simulink model "c221007_FCEV_CDCS"  (R2022b)
settings: Solver=ode4  StartTime=1  StopTime=size(Driving_cycle_v_kmph,1)  FixedStep=Auto  RelTol=1e-3  EnableMultiTasking=on
values from neighbouring files (symbols this model uses):
  Bat_eff_chg_average = 0.969    [FCEV_original_data.mat]
  Bat_eff_dis_average = 0.9632    [FCEV_original_data.mat]
  Bat_end_of_life_percent = 20    [FCEV_original_data.mat]
  Bat_I_chg_max = -120    [FCEV_original_data.mat]
  Bat_I_dis_max = 200    [FCEV_original_data.mat]
  Bat_nom_Ic = 2.5    [FCEV_original_data.mat]
  Bat_nom_SOC = 0.35    [FCEV_original_data.mat]
  Bat_nom_temp_oC = 25    [FCEV_original_data.mat]
  Bat_num_pa = 9    [FCEV_original_data.mat]
  Bat_num_se = 97    [FCEV_original_data.mat]
  Bat_ori_C1_chg_F = [397.526659684 455.660832136 435.08783522 460.845064365 457.605812374 417.289828504 416.373906992 359.741413056 321.561704819 1109.14132554 1165.67733205 1135.97600211 ... (72 elements, 9x8)]    [FCEV_original_data.mat]
  Bat_ori_C1_dis_F = [187.121968588 287.083505726 346.448009002 395.529439835 387.517274826 389.973134196 432.856765051 486.92921923 512.158935268 425.990733989 614.68708868 771.472592368 ... (72 elements, 9x8)]    [FCEV_original_data.mat]
  Bat_ori_C2_chg_F = [8748.48589695 7773.35875681 9404.86567646 8934.73981058 8290.58671366 7592.78422269 7759.44623103 7396.59043829 6151.35152293 16187.7227039 11721.8480541 13157.8579836 ... (72 elements, 9x8)]    [FCEV_original_data.mat]
  Bat_ori_C2_dis_F = [2939.81325553 4590.73311898 5504.93546413 5887.5077374 6534.37836712 7765.46899768 10584.7751706 10372.0508438 9238.72693885 5207.86390693 7911.43744944 8879.62137571 ... (72 elements, 9x8)]    [FCEV_original_data.mat]
  Bat_ori_cap_max_Ah = 20.7    [Config_c221218.m]    (also in Config_c230117.m; Config_c230321.m; FCEV_original_data.mat)
  Bat_ori_dUdt4 = [-0.303773584906 -0.249056603774 -0.115094339623 -0.0396226415094 0.0396226415094 0.0641509433962 0.107547169811 0.111320754717 0.0415094339623 0.0547169811321 0.130188679245]    [FCEV_original_data.mat]
  Bat_ori_R0_chg_O = [0.0771669453735 0.0731809311402 0.0726556782939 0.0729965156794 0.0731758310684 0.0742031005051 0.0721266921026 0.0714211058078 0.0714186176143 0.0374124505155 0.0354566732504 0.0345430657188 ... (72 elements, 9x8)]    [FCEV_original_data.mat]
  Bat_ori_R0_dis_O = [0.0819458671157 0.0812429476608 0.0803749674507 0.0805513601722 0.0838629023857 0.0850797840015 0.0829875518672 0.0826388888889 0.0812514106148 0.0428124986417 0.0424658903711 0.0428572670451 ... (72 elements, 9x8)]    [FCEV_original_data.mat]
  Bat_ori_R1_chg_O = [0.114339870884 0.105392753268 0.104421193553 0.109821896183 0.114868279838 0.123333154908 0.129174812826 0.149917249373 0.174896487845 0.0420560161846 0.0390948352938 0.0370122837364 ... (72 elements, 9x8)]    [FCEV_original_data.mat]
  Bat_ori_R1_dis_O = [0.304806399643 0.213604089624 0.171463520004 0.151183840498 0.140630862434 0.128795299077 0.116857791733 0.112567113582 0.106368362501 0.0943235089866 0.0730697254134 0.0611414736086 ... (72 elements, 9x8)]    [FCEV_original_data.mat]
  Bat_ori_R2_chg_O = [0.134518959939 0.17565045702 0.161100627268 0.189032232545 0.205639040497 0.226170473035 0.223651875822 0.181765694192 0.212966950836 0.073628872144 0.0788540822416 0.0792414571734 ... (72 elements, 9x8)]    [FCEV_original_data.mat]
  Bat_ori_R2_dis_O = [0.354968099904 0.285293035102 0.286338708953 0.298763853987 0.248762838155 0.178586175471 0.129047399775 0.188406991173 0.174494800676 0.131839238891 0.123225430215 0.132069033134 ... (72 elements, 9x8)]    [FCEV_original_data.mat]
  Bat_ori_SOC2 = [0 0.001 0.002 0.003 0.004 0.005 0.006 0.007 0.008 0.009 0.01 0.011 ... (1001 elements, 1x1001)]    [FCEV_original_data.mat]
  Bat_ori_SOC4 = [-0.00598301069999 0.0920117618231 0.190864167279 0.289083557951 0.387343788287 0.485011843502 0.5850485992 0.678163031937 0.774810095565 0.876684636119 0.972739524626]    [FCEV_original_data.mat]
  Bat_ori_Uoc_chg_V = [2.4478 2.54923264342 2.6007 2.6383 2.66953057366 2.69636321708 2.7197 2.74042850391 2.75906114733 2.77619379074 2.792 2.80675907757 ... (1001 elements, 1x1001)]    [FCEV_original_data.mat]
  Bat_ori_Uoc_dis_V = [1.9998 2.03916768329 2.24724374236 2.39700902919 2.48767431602 2.5476 2.5882 2.6202 2.64771773167 2.6719 2.6933 2.71251566192 ... (1001 elements, 1x1001)]    [FCEV_original_data.mat]
  Bat_ori_Uoc_V = [2.2238 2.29420016335 2.42397187118 2.5176545146 2.57860244484 2.62198160854 2.65395 2.68031425195 2.7033894395 2.72404689537 2.74265 2.75963736975 ... (1001 elements, 1x1001)]    [FCEV_original_data.mat]
  Bat_single_capacity_nom_Ah = 2.3    [FCEV_original_data.mat]
  Bat_SOC_cs_max = 0.4    [FCEV_original_data.mat]
  Bat_SOC_cs_min = 0.2    [FCEV_original_data.mat]
  Bat_SOC_ini = 0.3    [Config_c22100601.m]    (also in Config_c22100701.m; FCEV_original_data.mat = 0.45)
  Bat_SOC_max = 0.9    [FCEV_original_data.mat]
  Bat_SOC_min = 0.3    [FCEV_original_data.mat]
  Bat_temp_amb_oC = 25    [FCEV_original_data.mat]
  Bat_temp_cool_oC = 25    [FCEV_original_data.mat]
  Bat_U_avg_V = Bat_num_se*mean(Bat_ori_Uoc_V)    [Config_c22100601.m]    (also in Config_c22100701.m)
  DCAC_eff = 0.95    [FCEV_original_data.mat]
  DCDC_ori_eff = [0.95 0.96 0.97 0.976 0.98 0.978 0.973 0.962]    [FCEV_original_data.mat]
  DCDC_ori_power_kW = [0 10 20 30 40 50 60 70]    [FCEV_original_data.mat]
  FC_fuel_mass_ini_kg = 10    [FCEV_original_data.mat]
  FC_ori_eff = [0.1 0.33 0.492 0.533 0.559 0.596 0.591 0.562 0.508]    [FCEV_original_data.mat]
  FC_ori_fuel_rate_gps = [0 0.0505050505051 0.0846883468835 0.117260787992 0.149075730471 0.279642058166 0.423011844332 0.593119810202 0.820209973753]    [FCEV_original_data.mat]
  FC_ori_power_kW = [0 2 5 7.5 10 20 30 40 50]    [FCEV_original_data.mat]
  FC_power_max_kW = 50    [FCEV_original_data.mat]
  FC_power_min_kW = 0    [FCEV_original_data.mat]
  MC_eff_brk_average = 0.810578512397    [FCEV_original_data.mat]
  MC_eff_dri_average = 0.810578512397    [FCEV_original_data.mat]
  MC_inertia = 0.06    [FCEV_original_data.mat]
  MC_ori_eff = [0.7 0.78 0.85 0.86 0.81 0.82 0.79 0.78 0.78 0.78 0.78 0.7 ... (231 elements, 11x21)]    [FCEV_original_data.mat]
  MC_ori_power_brk_req_kW = [0 -28.3912930389 -56.7825860779 -85.1738791168 -113.565172156 -141.956465195 -170.347758234 -198.739051273 -227.130344311 -255.52163735 -283.912930389 0 ... (121 elements, 11x11)]    [FCEV_original_data.mat]
  MC_ori_power_dri_req_kW = [0 0 0 0 0 0 0 0 0 0 0 0 ... (121 elements, 11x11)]    [FCEV_original_data.mat]
  MC_ori_spd_rpm = [0 1000 2000 3000 4000 5000 6000 7000 8000 9000 10000]    [FCEV_original_data.mat]
  MC_ori_trq_brk_max_Nm = [-271.1368 -271.1368 -271.1368 -237.5159 -178.1369 -142.4824 -118.7579 -101.8119 -89.0685 -79.172 -71.1734]    [FCEV_original_data.mat]
  MC_ori_trq_brk_Nm = [-271.136848522 -244.02316367 -216.909478817 -189.795793965 -162.682109113 -135.568424261 -108.454739409 -81.3410545565 -54.2273697044 -27.1136848522 0]    [FCEV_original_data.mat]
  MC_ori_trq_dri_max_Nm = [271.1368 271.1368 271.1368 237.5159 178.1369 142.4824 118.7579 101.8119 89.0685 79.172 71.1734]    [FCEV_original_data.mat]
  MC_ori_trq_dri_Nm = [0 27.1136848522 54.2273697044 81.3410545565 108.454739409 135.568424261 162.682109113 189.795793965 216.909478817 244.02316367 271.136848522]    [FCEV_original_data.mat]
  MC_ori_trq_Nm = [-271.136848522 -244.02316367 -216.909478817 -189.795793965 -162.682109113 -135.568424261 -108.454739409 -81.3410545565 -54.2273697044 -27.1136848522 0 27.1136848522 ... (21 elements, 1x21)]    [FCEV_original_data.mat]
  MC_power_max_kW = 75    [FCEV_original_data.mat]
  MC_spd_max_rpm = 10000    [FCEV_original_data.mat]
  MC_spd_min_rpm = 0    [FCEV_original_data.mat]
  MC_spd_scale = 1    [FCEV_original_data.mat]
  MC_trq_scale = 1    [FCEV_original_data.mat]
  MC_U_min_V = 120    [FCEV_original_data.mat]
  Road_u = 0.75    [FCEV_original_data.mat]
  S_r = floor(max(Sr_SOC_process(:,1))):-1:0    [Config_c22100601.m]    (also in Config_c22100701.m)
  Time_sample = 60    [Driving_cycle_recognition_data.mat]
  Trip_distance_total_km = sum(Driving_cycle_v_kmph(:,2)/3.6)/1000    [Config_c22100601.m]    (also in Config_c22100701.m)
  usd2rmb = 7.116    [Config_c22100601.m]    (also in Config_c22100701.m; Config_c221106.m = 6; Config_c221112.m = 6; Config_c221127.m = 6)
  Veh_air_density_kgpm2 = 1.2    [FCEV_original_data.mat]
  Veh_brk_front = [1 0.6 0.608 0.61 0.618 0.624 0.636 0.645 0.655]    [FCEV_original_data.mat]
  Veh_brk_z = [0.1 0.2 0.3 0.4 0.5 0.6 0.7 0.8 0.9]    [FCEV_original_data.mat]
  Veh_brk_z_max = 0.7    [FCEV_original_data.mat]
  Veh_brk_z_min = 0.1    [FCEV_original_data.mat]
  Veh_coeff_drag = 0.312    [FCEV_original_data.mat]
  Veh_coeff_roll = 0.00863    [FCEV_original_data.mat]
  Veh_final_drive_inertia = 0.1105    [FCEV_original_data.mat]
  Veh_final_drive_ratio = 3.47    [FCEV_original_data.mat]
  Veh_frontal_area_m2 = 2.06    [FCEV_original_data.mat]
  Veh_gravity_acc_ms2 = 9.81    [FCEV_original_data.mat]
  Veh_mass_cargo_kg = 113    [FCEV_original_data.mat]
  Veh_mass_curb_kg = 1157    [FCEV_original_data.mat]
  Veh_mech_eff = 0.9    [FCEV_original_data.mat]
  Veh_rotary_mass_conversion_factor = 1.05    [FCEV_original_data.mat]
  Veh_size_cg_height_m = 0.53    [FCEV_original_data.mat]
  Veh_wheel_inertia = 3.1039    [FCEV_original_data.mat]
  Veh_wheel_radius_m = 0.313    [FCEV_original_data.mat]
  Veh_wt_frac_front = 0.5    [FCEV_original_data.mat]
undefined symbols (not defined in the file or in its folder): alpha, Bat_ori_temp, Sr_e
libraries: neural x10
(part 2 of 5)

== system c221007_FCEV_CDCS/整车动力学模型/加速阻力 ==
  车速 km/h : Inport
  Add : Sum  Inputs=+-
  Add1 : Sum  Inputs=+-
  Add2 : Sum
  Clock : Clock
  Constant : Constant  Value=0
  Constant1 : Constant  Value=Veh_rotary_mass_conversion_factor
  Constant2 : Constant  Value=Veh_mass_curb_kg
  Constant3 : Constant  Value=Veh_mass_cargo_kg
  Divide : Product  Inputs=***/
  Fj : Scope
  Gain : Gain
  Memory : Memory  InheritSampleTime=on
  Memory1 : Memory
  Saturation : Saturate  UpperLimit=1.1  LowerLimit=0.9
  Switch : Switch  Criteria=u2 > Threshold  SaturateOnIntegerOverflow=off  InputSameDT=off
  km/h->m/s : Gain  Gain=1/3.6
  加速阻力 N : Outport
  wires:
  车速 km/h/1 -> Memory/1, Add/1
  Add/1 -> km/h->m/s/1
  km/h->m/s/1 -> Switch/2, Divide/2
  Gain/1 -> 加速阻力 N/1, Fj/1
  Memory/1 -> Add/2
  Memory1/1 -> Add1/2
  Add2/1 -> Divide/1
  Constant2/1 -> Add2/1
  Constant3/1 -> Add2/2
  Constant1/1 -> Divide/3
  Clock/1 -> Memory1/1, Add1/1
  Divide/1 -> Switch/1
  Constant/1 -> Switch/3
  Switch/1 -> Gain/1
  Add1/1 -> Saturation/1
  Saturation/1 -> Divide/4

== system c221007_FCEV_CDCS/整车动力学模型/坡道阻力 ==
  车辆平均车速1 : Inport
  预测坡度 : Inport  Port=2
  Add : Sum  Inputs=+-
  Add1 : Sum
  Constant : Constant  Value=0
  Constant1 : Constant  Value=Veh_mass_cargo_kg
  Constant2 : Constant  Value=Veh_mass_curb_kg
  Constant3 : Constant  Value=Veh_gravity_acc_ms2
  Fi : Scope
  Memory : Memory  InheritSampleTime=on
  Product : Product  Inputs=3  RndMeth=Zero
  Switch : Switch  SaturateOnIntegerOverflow=off  InputSameDT=off
  Switch1 : Switch  Criteria=u2 > Threshold  SaturateOnIntegerOverflow=off  InputSameDT=off
  Trigonometric Function : Trigonometry  Operator=atan
  Trigonometric Function1 : Trigonometry
  坡道阻力 N : Outport
  wires:
  Trigonometric Function/1 -> Trigonometric Function1/1
  Trigonometric Function1/1 -> Product/1
  Constant3/1 -> Product/3
  Constant/1 -> Switch/3, Switch1/3
  预测坡度/1 -> Trigonometric Function/1
  Switch1/1 -> 坡道阻力 N/1, Fi/1
  Add1/1 -> Product/2
  Constant2/1 -> Add1/1
  Constant1/1 -> Add1/2
  车辆平均车速1/1 -> Add/1, Memory/1, Switch1/2
  Memory/1 -> Add/2
  Product/1 -> Switch/1
  Add/1 -> Switch/2
  Switch/1 -> Switch1/1

== system c221007_FCEV_CDCS/整车动力学模型/滚动阻力 ==
  车辆平均车速 km/h : Inport
  预测坡度 : Inport  Port=2
  "  1" : Constant  Value=Veh_coeff_roll
  Add : Sum  Inputs=+-
  Add1 : Sum
  Constant : Constant  Value=0
  Constant1 : Constant  Value=Veh_gravity_acc_ms2
  Constant2 : Constant  Value=Veh_mass_curb_kg
  Constant3 : Constant  Value=Veh_mass_cargo_kg
  Fcn1 : Fcn  Expr=atan(u)
  Fcn2 : Fcn  Expr=cos(u)
  Ff : Scope
  Memory : Memory  InheritSampleTime=on
  Product : Product  Inputs=4  RndMeth=Zero
  Switch : Switch  Criteria=u2 > Threshold  SaturateOnIntegerOverflow=off  InputSameDT=off
  Switch1 : Switch  SaturateOnIntegerOverflow=off  InputSameDT=off
  滚动阻力 N : Outport
  wires:
  Fcn2/1 -> Product/3
  Constant/1 -> Switch1/3, Switch/3
  Add1/1 -> Product/1
  Fcn1/1 -> Fcn2/1
  预测坡度/1 -> Fcn1/1
  Constant2/1 -> Add1/1
  Constant3/1 -> Add1/2
  车辆平均车速 km/h/1 -> Switch/2, Memory/1, Add/1
  Switch/1 -> Ff/1, 滚动阻力 N/1
  Constant1/1 -> Product/2
  "  1"/1 -> Product/4
  Product/1 -> Switch1/1
  Memory/1 -> Add/2
  Add/1 -> Switch1/2
  Switch1/1 -> Switch/1

== system c221007_FCEV_CDCS/整车动力学模型/空气阻力 ==
  veh_spd km/h : Inport
  Add : Sum  Inputs=-+
  Constant : Constant  Value=0
  Constant1 : Constant  Value=Veh_frontal_area_m2
  Constant2 : Constant  Value=Veh_coeff_drag
  Fw : Scope
  Gain : Gain  Gain=1/21.15
  Memory : Memory  InheritSampleTime=on
  Product : Product  Inputs=4  RndMeth=Zero
  Switch : Switch  SaturateOnIntegerOverflow=off  InputSameDT=off
  空气阻力 N : Outport
  wires:
  Constant1/1 -> Product/1
  Constant2/1 -> Product/2
  veh_spd km/h/1 -> Product/3, Memory/1, Add/2, Product/4
  Product/1 -> Gain/1
  Constant/1 -> Switch/3
  Gain/1 -> Switch/1
  Add/1 -> Switch/2
  Memory/1 -> Add/1
  Switch/1 -> Fw/1, 空气阻力 N/1

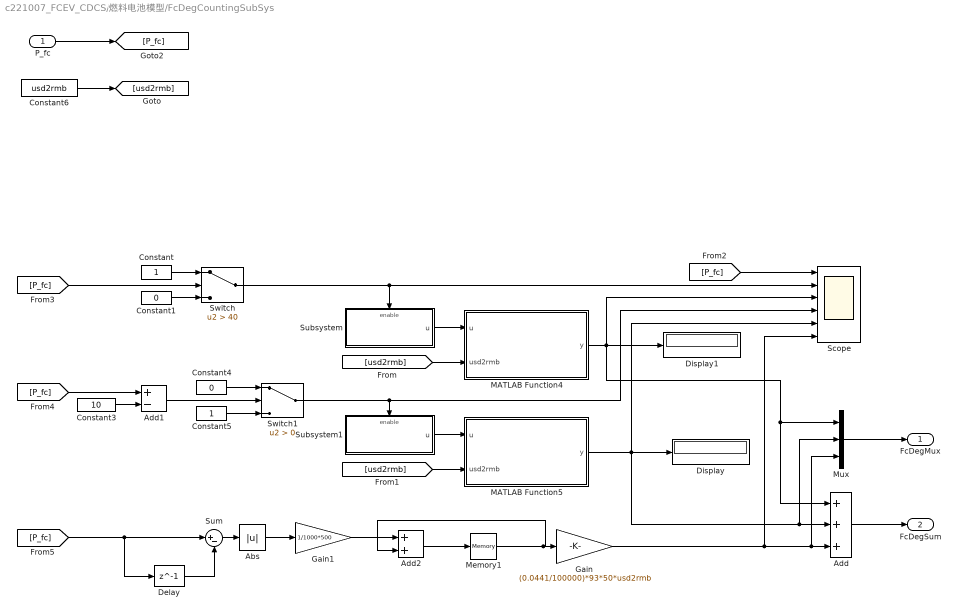
== system c221007_FCEV_CDCS/燃料电池模型/FcDegCountingSubSys ==
  P_fc : Inport
  Abs : Abs  SaturateOnIntegerOverflow=off
  Add : Sum  Inputs=+++
  Add1 : Sum  Inputs=+-
  Add2 : Sum
  Constant : Constant
  Constant1 : Constant  Value=0
  Constant3 : Constant  Value=10
  Constant4 : Constant  Value=0
  Constant5 : Constant
  Constant6 : Constant  Value=usd2rmb
  Delay : Delay  DelayLength=1
  Display : Display
  Display1 : Display
  Gain : Gain  Gain=(0.0441/100000)*93*50*usd2rmb
  Gain1 : Gain  Gain=1/1000*500
  MATLAB Function4 : MATLAB Function  TreatAsAtomicUnit=on
  MATLAB Function5 : MATLAB Function  TreatAsAtomicUnit=on
  Memory1 : Memory
  Mux : Mux  Inputs=3
  Scope : Scope  NumInputPorts=6
  Subsystem : Subsystem
  Subsystem1 : Subsystem
  Sum : Sum  Inputs=|+-
  Switch : Switch  Criteria=u2 > Threshold  Threshold=40  SaturateOnIntegerOverflow=off  InputSameDT=off
  Switch1 : Switch  Criteria=u2 > Threshold  SaturateOnIntegerOverflow=off  InputSameDT=off
  FcDegMux : Outport
  FcDegSum : Outport  Port=2
  wires:
  MATLAB Function5/1(y) -> Scope/5, Display/1, Mux/2, Add/2
  Constant3/1 -> Add1/2
  Constant5/1 -> Switch1/3
  Switch1/1 -> Scope/4, Subsystem1/Enable
  Add1/1 -> Switch1/2
  Subsystem/1(u) -> MATLAB Function4/1(u)
  Constant/1 -> Switch/1
  [usd2rmb] -> MATLAB Function4/2(usd2rmb)
  Constant1/1 -> Switch/3
  Constant4/1 -> Switch1/1
  [usd2rmb] -> MATLAB Function5/2(usd2rmb)
  Switch/1 -> Scope/2, Subsystem/Enable
  P_fc/1 -> [P_fc]
  Subsystem1/1(u) -> MATLAB Function5/1(u)
  MATLAB Function4/1(y) -> Scope/3, Mux/1, Add/1, Display1/1
  Constant6/1 -> [usd2rmb]
  [P_fc] -> Scope/1
  Gain/1 -> Scope/6, Mux/3, Add/3
  Gain1/1 -> Add2/1
  Add2/1 -> Memory1/1
  Sum/1 -> Abs/1
  Abs/1 -> Gain1/1
  Delay/1 -> Sum/2
  Memory1/1 -> Gain/1, Add2/2
  [P_fc] -> Delay/1, Sum/1
  [P_fc] -> Switch/2
  [P_fc] -> Add1/1
  Add/1 -> FcDegSum/1
  Mux/1 -> FcDegMux/1

== system c221007_FCEV_CDCS/燃料电池模型/Fuel Rate Calculation1 ==
  note: Transient load response
  fc pwr : Inport
  "FC hydrogen consumption rate " : Lookup_n-D  NumberOfTableDimensions=1  BreakpointsForDimension1=FC_ori_power_kW  Table=FC_ori_fuel_rate_gps  RndMeth=Simplest
  fcv_H2_rate (g/s)1 : Outport
  wires:
  fc pwr/1 -> "FC hydrogen consumption rate "/1
  "FC hydrogen consumption rate "/1 -> fcv_H2_rate (g/s)1/1  "fcv_hot_H2_hist"

== system c221007_FCEV_CDCS/燃料电池模型/Fuel cell efficiency calculation ==
  note: Transient load response
  fc power : Inport
  "FC efficiency " : Lookup_n-D  NumberOfTableDimensions=1  BreakpointsForDimension1=FC_ori_power_kW  Table=FC_ori_eff  RndMeth=Simplest
  "fc_eff " : Outport
  wires:
  "FC efficiency "/1 -> "fc_eff "/1
  fc power/1 -> "FC efficiency "/1

== system c221007_FCEV_CDCS/燃料电池模型/Power Calculation ==
  note: Transient load response
  fc on : Inport
  Power command (kW) : Inport  Port=2
  "   " : Constant  Value=0
  Switch2 : Switch  Threshold=0.5
  Power output (kW) : Outport
  wires:
  "   "/1 -> Switch2/3
  Power command (kW)/1 -> Switch2/1
  fc on/1 -> Switch2/2
  Switch2/1 -> Power output (kW)/1

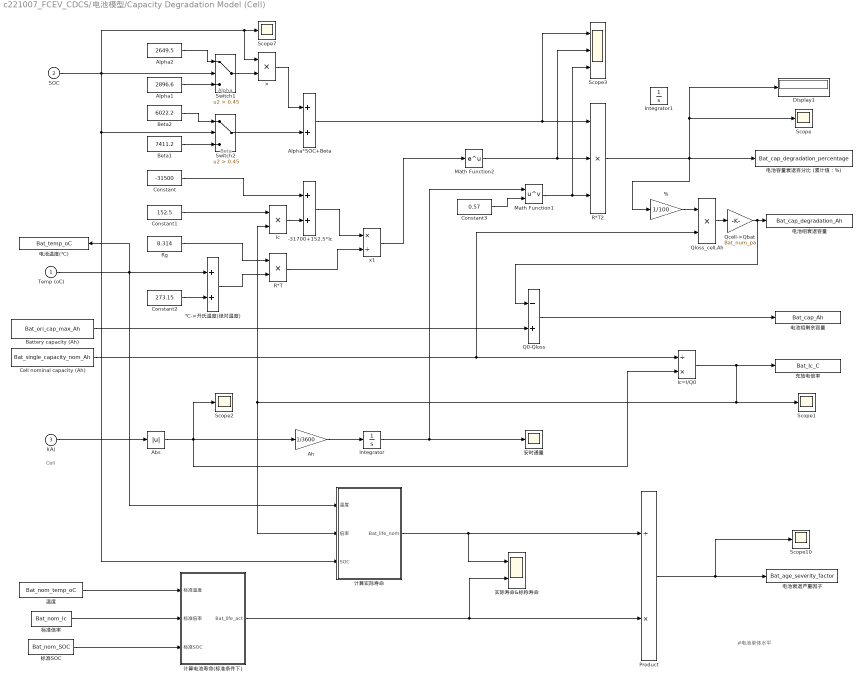
== system c221007_FCEV_CDCS/电池模型/Capacity Degradation Model (Cell) ==
  note: Cell
  note: #电池单体水平
  note: Beta
  note: Alpha
  Temp (oC) : Inport
  SOC : Inport  Port=2
  I(A) : Inport  Port=3
  % : Gain  Gain=1/100
  -31700+152.5*Ic : Sum  InputSameDT=on  SaturateOnIntegerOverflow=on  OutDataTypeStr=Inherit: Same as first input
  Abs : Abs  SaturateOnIntegerOverflow=off
  Ah : Gain  Gain=1/3600
  Alpha*SOC+Beta : Sum  InputSameDT=on  SaturateOnIntegerOverflow=on  OutDataTypeStr=Inherit: Same as first input
  Alpha1 : Constant  Value=2896.6
  Alpha2 : Constant  Value=2649.5
  Battery capacity (Ah) : Constant  Value=Bat_ori_cap_max_Ah
  Beta1 : Constant  Value=7411.2
  Beta2 : Constant  Value=6022.2
  Cell nominal capacity (Ah) : Constant  Value=Bat_single_capacity_nom_Ah
  Constant : Constant  Value=-31500
  Constant1 : Constant  Value=152.5
  Constant2 : Constant  Value=273.15
  Constant3 : Constant  Value=0.57
  Display1 : Display
  Ic : Product  InputSameDT=on  RndMeth=Zero  SaturateOnIntegerOverflow=on  OutDataTypeStr=Inherit: Same as first input
  Ic=I/Q0 : Product  Inputs=/*  InputSameDT=on  RndMeth=Zero  SaturateOnIntegerOverflow=on  OutDataTypeStr=Inherit: Same as first input
  Integrator : Integrator  InitialCondition=eps
  Integrator1 : Integrator
  Math Function1 : Math  Operator=pow  SignedPower=on
  Math Function2 : Math  SignedPower=on
  Product : Product  Inputs=/*
  Q0-Qloss : Sum  Inputs=-+  InputSameDT=on  SaturateOnIntegerOverflow=on  OutDataTypeStr=Inherit: Same as first input
  Qcell->Qbat : Gain  Gain=Bat_num_pa  SaturateOnIntegerOverflow=on  OutDataTypeStr=Inherit: Same as input  ParamDataTypeStr=Inherit: Same as input
  Qloss_cell,Ah : Product  InputSameDT=on  RndMeth=Zero  SaturateOnIntegerOverflow=on  OutDataTypeStr=Inherit: Same as first input
  R*T : Product  InputSameDT=on  RndMeth=Zero  SaturateOnIntegerOverflow=on  OutDataTypeStr=Inherit: Same as first input
  R*T2 : Product  Inputs=3  InputSameDT=on  RndMeth=Zero  SaturateOnIntegerOverflow=on  OutDataTypeStr=Inherit: Same as first input
  Rg : Constant  Value=8.314
  Scope{,1..2,7,10} (5 alike) : Scope
  Scope3 : Scope  NumInputPorts=3
  Switch1 : Switch  Criteria=u2 > Threshold  Threshold=0.45
  Switch2 : Switch  Criteria=u2 > Threshold  Threshold=0.45
  x1 : Product  Inputs=*/  InputSameDT=on  RndMeth=Zero  SaturateOnIntegerOverflow=on  OutDataTypeStr=Inherit: Same as first input
  × : Product  InputSameDT=on  RndMeth=Zero  SaturateOnIntegerOverflow=on  OutDataTypeStr=Inherit: Same as first input
  ℃->开氏温度(绝对温度) : Sum  InputSameDT=on  SaturateOnIntegerOverflow=on  OutDataTypeStr=Inherit: Same as first input
  充放电倍率 : ToWorkspace  VariableName=Bat_Ic_C  SampleTime=-1
  安时通量 : Scope
  实际寿命&标称寿命 : Scope  NumInputPorts=2
  标准SOC : Constant  Value=Bat_nom_SOC
  标准倍率 : Constant  Value=Bat_nom_Ic
  温度 : Constant  Value=Bat_nom_temp_oC  VectorParams1D=off
  电池容量衰退百分比 (累计值：%) : ToWorkspace  VariableName=Bat_cap_degradation_percentage  SampleTime=-1
  电池温度(℃) : ToWorkspace  VariableName=Bat_temp_oC  SampleTime=-1
  电池组剩余容量 : ToWorkspace  VariableName=Bat_cap_Ah  SampleTime=-1
  电池组衰退容量 : ToWorkspace  VariableName=Bat_cap_degradation_Ah  SampleTime=-1
  电池衰退严重因子 : ToWorkspace  VariableName=Bat_age_severity_factor  SampleTime=-1
  计算实际寿命 : Subsystem
  计算电池寿命(标准条件下) : Subsystem
  wires:
  SOC/1 -> Switch1/2, Scope7/1, ×/1, Switch2/2, 计算实际寿命/3(SOC)
  Alpha2/1 -> Switch1/1
  Alpha1/1 -> Switch1/3
  Beta2/1 -> Switch2/1
  Beta1/1 -> Switch2/3
  Switch1/1 -> ×/2
  Switch2/1 -> Alpha*SOC+Beta/2
  ×/1 -> Alpha*SOC+Beta/1
  Rg/1 -> R*T/1
  ℃->开氏温度(绝对温度)/1 -> R*T/2
  Ic=I/Q0/1 -> Scope1/1, Ic/2, 计算实际寿命/2(倍率), 充放电倍率/1
  Alpha*SOC+Beta/1 -> R*T2/1, Scope3/1
  Constant/1 -> -31700+152.5*Ic/1
  Ic/1 -> -31700+152.5*Ic/2
  Constant1/1 -> Ic/1
  -31700+152.5*Ic/1 -> x1/1
  R*T/1 -> x1/2
  Math Function2/1 -> R*T2/2, Scope3/2
  x1/1 -> Math Function2/1
  Math Function1/1 -> R*T2/3, Scope3/3
  R*T2/1 -> Scope/1, Display1/1, 电池容量衰退百分比 (累计值：%)/1, %/1
  Abs/1 -> Ic=I/Q0/2, Ah/1, Scope2/1
  Integrator/1 -> Math Function1/1, 安时通量/1
  Temp (oC)/1 -> 计算实际寿命/1(温度), 电池温度(℃)/1, ℃->开氏温度(绝对温度)/1
  Constant2/1 -> ℃->开氏温度(绝对温度)/2
  %/1 -> Qloss_cell,Ah/1
  温度/1 -> 计算电池寿命(标准条件下)/1(标准温度)
  标准倍率/1 -> 计算电池寿命(标准条件下)/2(标准倍率)
  标准SOC/1 -> 计算电池寿命(标准条件下)/3(标准SOC)
  Product/1 -> 电池衰退严重因子/1, Scope10/1
  计算实际寿命/1(Bat_life_nom) -> 实际寿命&标称寿命/1, Product/1
  计算电池寿命(标准条件下)/1(Bat_life_act) -> Product/2, 实际寿命&标称寿命/2
  I(A)/1 -> Abs/1
  Cell nominal capacity (Ah)/1 -> Qloss_cell,Ah/2, Ic=I/Q0/1
  Qcell->Qbat/1 -> Q0-Qloss/1, 电池组衰退容量/1
  Qloss_cell,Ah/1 -> Qcell->Qbat/1
  Battery capacity (Ah)/1 -> Q0-Qloss/2
  Q0-Qloss/1 -> 电池组剩余容量/1
  Ah/1 -> Integrator/1
  Constant3/1 -> Math Function1/2

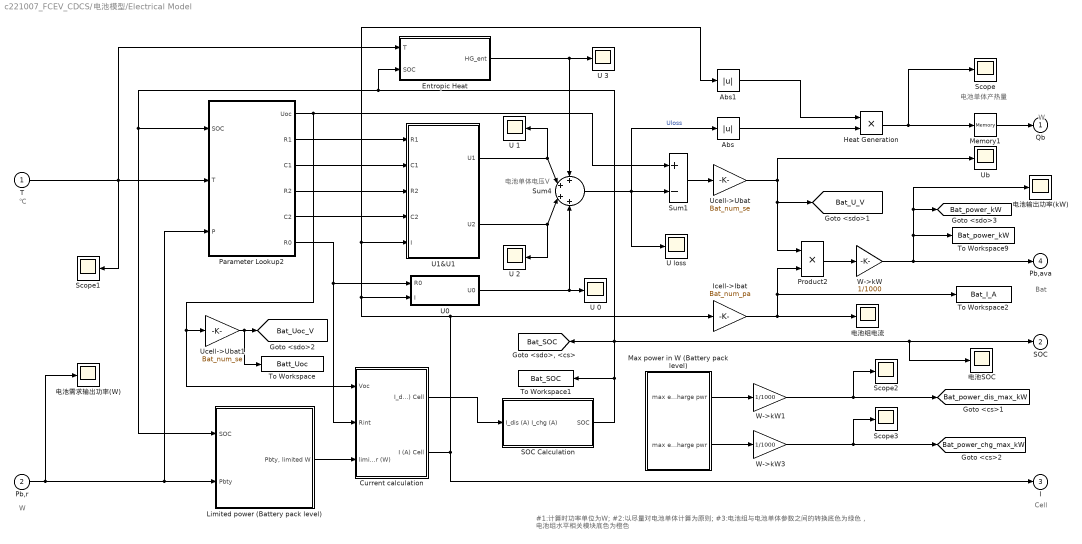
== system c221007_FCEV_CDCS/电池模型/Electrical Model ==
  note: Bat
  note: Cell
  note: W
  note: ℃
  note: #1:计算时功率单位为W;
      | #2:以尽量对电池单体计算为原则;
      | #3:电池组与电池单体参数之间的转换底色为绿色， 电池组水平相关模块底色为橙色
  note: W
  note: 电池单体产热量
  note: 电池单体电压V
  T : Inport
  Pb,r : Inport  Port=2
  Abs : Abs  SaturateOnIntegerOverflow=off
  Abs1 : Abs  SaturateOnIntegerOverflow=off
  Current calculation : Subsystem
  Entropic Heat : Subsystem
  Heat Generation : Product  RndMeth=Zero
  Icell->Ibat : Gain  Gain=Bat_num_pa  SaturateOnIntegerOverflow=on  OutDataTypeStr=Inherit: Same as input  ParamDataTypeStr=Inherit: Same as input
  Limited power (Battery pack level) : Subsystem
  Max power in W (Battery pack level) : Subsystem
  Memory1 : Memory  InheritSampleTime=on
  Parameter Lookup2 : Subsystem
  Product2 : Product  RndMeth=Zero
  SOC Calculation : Subsystem
  Scope{,1..3} (4 alike) : Scope
  Sum1 : Sum  Inputs=+-
  Sum4 : Sum  Inputs=++++
  To Workspace : ToWorkspace  VariableName=Batt_Uoc  SaveFormat=Timeseries  SampleTime=-1
  To Workspace1 : ToWorkspace  VariableName=Bat_SOC  SampleTime=-1
  To Workspace2 : ToWorkspace  VariableName=Bat_I_A  SampleTime=-1
  To Workspace9 : ToWorkspace  VariableName=Bat_power_kW  SampleTime=-1
  U {0..3} (4 alike) : Scope
  U loss : Scope
  U0 : Subsystem
  U1&U1 : Subsystem
  Ub : Scope
  Ucell->Ubat : Gain  Gain=Bat_num_se  SaturateOnIntegerOverflow=on  OutDataTypeStr=Inherit: Same as input  ParamDataTypeStr=Inherit: Same as input
  Ucell->Ubat1 : Gain  Gain=Bat_num_se  SaturateOnIntegerOverflow=on  OutDataTypeStr=Inherit: Same as input  ParamDataTypeStr=Inherit: Same as input
  W->kW : Gain  Gain=1/1000  SaturateOnIntegerOverflow=on  OutDataTypeStr=Inherit: Same as input  ParamDataTypeStr=Inherit: Same as input
  W->kW1 : Gain  Gain=1/1000  SaturateOnIntegerOverflow=on  OutDataTypeStr=Inherit: Same as input  ParamDataTypeStr=Inherit: Same as input
  W->kW3 : Gain  Gain=1/1000  SaturateOnIntegerOverflow=on  OutDataTypeStr=Inherit: Same as input  ParamDataTypeStr=Inherit: Same as input
  电池SOC : Scope
  电池组电流 : Scope
  电池输出功率(kW) : Scope
  电池需求输出功率(W) : Scope
  Qb : Outport  InitialOutput=0
  SOC : Outport  Port=2  InitialOutput=0
  I : Outport  Port=3  InitialOutput=0
  Pb,ava : Outport  Port=4  InitialOutput=0
  tag scope: Bat_SOC=global, Bat_U_V=global, Bat_Uoc_V=global, Bat_power_chg_max_kW=global, Bat_power_dis_max_kW=global, Bat_power_kW=global
  wires:
  Parameter Lookup2/2(R1) -> U1&U1/1(R1)
  Parameter Lookup2/3(C1) -> U1&U1/2(C1)
  Parameter Lookup2/4(R2) -> U1&U1/3(R2)
  Parameter Lookup2/5(C2) -> U1&U1/4(C2)
  Parameter Lookup2/6(R0) -> U0/1(R0), Current calculation/2(Rint)
  U1&U1/1(U1) -> Sum4/2, U 1/1
  U1&U1/2(U2) -> U 2/1, Sum4/3
  Ucell->Ubat/1 -> Product2/1, [Bat_U_V], Ub/1
  Entropic Heat/1(HG_ent) -> U 3/1, Sum4/1
  Product2/1 -> W->kW/1
  W->kW/1 -> 电池输出功率(kW)/1, [Bat_power_kW], To Workspace9/1, Pb,ava/1
  Memory1/1 -> Qb/1
  Heat Generation/1 -> Scope/1, Memory1/1
  Current calculation/1(I_dis (A) I_chg (A) Cell) -> SOC Calculation/1(I_dis (A) I_chg (A))
  T/1 -> Scope1/1, Entropic Heat/1(T), Parameter Lookup2/2(T)
  Pb,r/1 -> 电池需求输出功率(W)/1, Limited power (Battery pack level)/2(Pbty), Parameter Lookup2/3(P)
  Icell->Ibat/1 -> Product2/2, To Workspace2/1, 电池组电流/1
  W->kW1/1 -> Scope2/1, [Bat_power_dis_max_kW]
  W->kW3/1 -> Scope3/1, [Bat_power_chg_max_kW]
  Max power in W (Battery pack level)/1(max ess discharge pwr) -> W->kW1/1
  Max power in W (Battery pack level)/2(max ess charge pwr) -> W->kW3/1
  Parameter Lookup2/1(Uoc) -> Sum1/1, Ucell->Ubat1/1, Current calculation/1(Voc)
  Ucell->Ubat1/1 -> To Workspace/1, [Bat_Uoc_V]
  Limited power (Battery pack level)/1("Pbty, limited W") -> Current calculation/3(limited output power (W))
  SOC Calculation/1(SOC) -> 电池SOC/1, SOC/1, [Bat_SOC], Entropic Heat/2(SOC), Limited power (Battery pack level)/1(SOC), Parameter Lookup2/1(SOC), To Workspace1/1
  Current calculation/2(I (A) Cell) -> Abs1/1, U1&U1/5(I), U0/2(I), Icell->Ibat/1, I/1
  U0/1(U0) -> U 0/1, Sum4/4
  Sum4/1 -> U loss/1, Abs/1, Sum1/2  "Uloss"
  Sum1/1 -> Ucell->Ubat/1
  Abs/1 -> Heat Generation/2
  Abs1/1 -> Heat Generation/1

== system c221007_FCEV_CDCS/电池模型/Subsystem ==
  note: Thermal Model (Cell)
  note: Electrical Model
  power req'd into bus (kW)1 : Inport
  Capacity Degradation Model (Cell)1 : Subsystem
  Electrical Model1 : Subsystem  Tag=electrical
  Gain1 : Gain  Gain=0.5
  Thermal Model1 : Subsystem
  Ts+Tc(℃)1 : Sum
  kW->W1 : Gain  Gain=1000  SaturateOnIntegerOverflow=on  OutDataTypeStr=Inherit: Same as input  ParamDataTypeStr=Inherit: Same as input
  温度(℃)1 : Scope
  电池需求输出功率(kW)1 : Scope
  输出功率(kW)1 : Scope
  Pb,ava1 : Outport  InitialOutput=0
  wires:
  Gain1/1 -> Electrical Model1/1(T), 温度(℃)1/1, Capacity Degradation Model (Cell)1/1(Temp (oC))
  power req'd into bus (kW)1/1 -> 电池需求输出功率(kW)1/1, kW->W1/1
  Ts+Tc(℃)1/1 -> Gain1/1
  kW->W1/1 -> Electrical Model1/2(Pb,r)
  Thermal Model1/1(Tc.) -> Ts+Tc(℃)1/1
  Electrical Model1/4(Pb,ava) -> Pb,ava1/1, 输出功率(kW)1/1
  Electrical Model1/1(Qb) -> Thermal Model1/1(Qb)
  Thermal Model1/2(Ts.) -> Ts+Tc(℃)1/2
  Electrical Model1/2(SOC) -> Capacity Degradation Model (Cell)1/2(SOC)
  Electrical Model1/3(I) -> Capacity Degradation Model (Cell)1/3(I(A))

== system c221007_FCEV_CDCS/电池模型/Thermal Model ==
  note: 需要设置温度初始值
  note: W
  note: Tf
  note: (k)
  note: 冷却液温度 ℃
  note: ℃
  note: ℃
  Qb : Inport
  (1-1/RsCs-1/RcCs)*Ts(k-1) : Product  Inputs=**  RndMeth=Zero
  (RC*Cc-1)*Tc(k-1)/RcCc : Product  Inputs=**  RndMeth=Zero
  (RC*Cc-1)/RcCc : Product  Inputs=*/  RndMeth=Zero
  Calculation : Subsystem
  Constant : Constant  Value=273
  Constant3 : Constant
  Math Function : Math  Operator=reciprocal  SignedPower=on
  Math Function1 : Math  Operator=reciprocal  SignedPower=on
  Qb(k-1)/Cc : Product  Inputs=*/  RndMeth=Zero
  Sum10 : Sum  Inputs=+++
  Sum11 : Sum  Inputs=+--|
  Sum3 : Sum  Inputs=+++
  Sum4 : Sum  Inputs=+-|
  Sum5 : Sum  Inputs=|+-
  Sum7 : Sum  Inputs=++|
  Sum9 : Sum  Inputs=-+|
  Tc (K) : Scope
  Tc (℃) : Scope
  Tc(k-1) : Memory  InitialCondition=Bat_temp_amb_oC+273.15  InheritSampleTime=on
  Tc(k-1)/RcCs : Product  Inputs=*/  RndMeth=Zero
  Tf/RsCs : Product  Inputs=*/  RndMeth=Zero
  Tf1 : Constant  Value=Bat_temp_cool_oC
  Ts (K) : Scope
  Ts (℃) : Scope
  Ts(k-1) : Memory  InitialCondition=Bat_temp_amb_oC+273.15  InheritSampleTime=on
  Ts(k-1)/RcCc : Product  Inputs=*/  RndMeth=Zero
  Tc. : Outport
  Ts. : Outport  Port=2
  wires:
  Calculation/1(Cc) -> Qb(k-1)/Cc/2
  Calculation/2(RcCc) -> (RC*Cc-1)/RcCc/2, Ts(k-1)/RcCc/2, Sum4/1
  Constant3/1 -> Sum11/1, Sum4/2
  Sum4/1 -> (RC*Cc-1)/RcCc/1
  Qb(k-1)/Cc/1 -> Sum3/1
  Ts(k-1)/RcCc/1 -> Sum3/2
  Tf1/1 -> Sum7/2
  Calculation/3(RsCs) -> Tf/RsCs/2, Math Function/1
  Sum7/1 -> Tf/RsCs/1
  Tf/RsCs/1 -> Sum10/1
  Calculation/4(RcCs) -> Tc(k-1)/RcCs/2, Math Function1/1
  Math Function1/1 -> Sum11/2
  Math Function/1 -> Sum11/3
  (1-1/RsCs-1/RcCs)*Ts(k-1)/1 -> Sum10/2
  Sum11/1 -> (1-1/RsCs-1/RcCs)*Ts(k-1)/1
  Tc(k-1)/RcCs/1 -> Sum10/3
  Sum3/1 -> Sum5/1, Tc(k-1)/1, Tc (K)/1
  Constant/1 -> Sum9/1, Sum5/2, Sum7/1
  Sum5/1 -> Tc (℃)/1, Tc./1
  Sum10/1 -> Sum9/2, Ts(k-1)/1, Ts (K)/1
  Sum9/1 -> Ts./1, Ts (℃)/1
  Ts(k-1)/1 -> Ts(k-1)/RcCc/1, (1-1/RsCs-1/RcCs)*Ts(k-1)/2
  (RC*Cc-1)*Tc(k-1)/RcCc/1 -> Sum3/3
  (RC*Cc-1)/RcCc/1 -> (RC*Cc-1)*Tc(k-1)/RcCc/1
  Tc(k-1)/1 -> Tc(k-1)/RcCs/1, (RC*Cc-1)*Tc(k-1)/RcCc/2
  Qb/1 -> Qb(k-1)/Cc/1

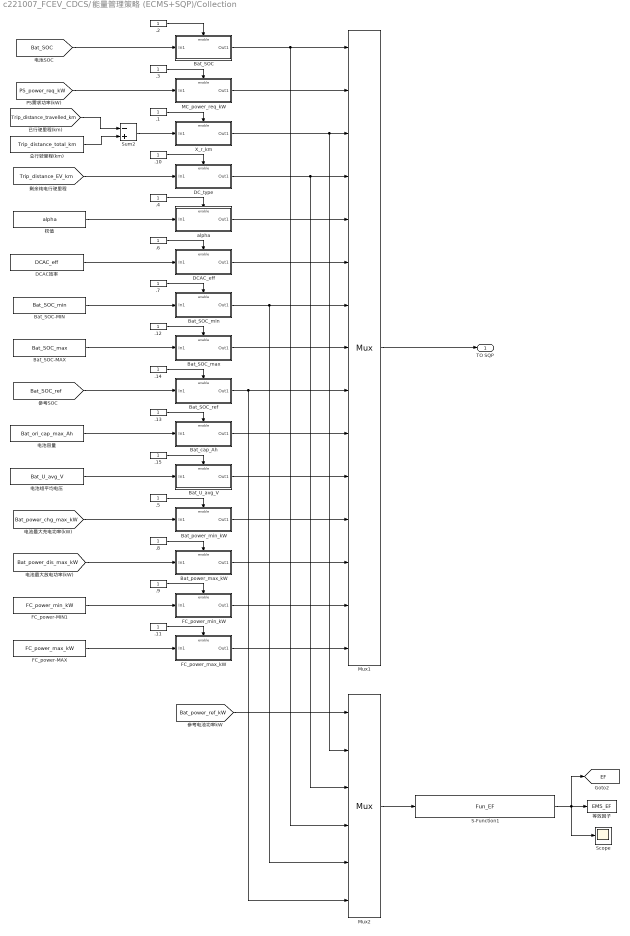
== system c221007_FCEV_CDCS/能量管理策略 (ECMS+SQP)/Collection ==
  "    DC_type" : Subsystem  TreatAsAtomicUnit=on
  .{1..15} (15 alike) : Constant
  Bat_SOC : Subsystem  TreatAsAtomicUnit=on
  Bat_SOC-MAX : Constant  Value=Bat_SOC_max
  Bat_SOC-MIN : Constant  Value=Bat_SOC_min
  Bat_SOC_max : Subsystem  TreatAsAtomicUnit=on
  Bat_SOC_min : Subsystem  TreatAsAtomicUnit=on
  Bat_SOC_ref : Subsystem  TreatAsAtomicUnit=on
  Bat_U_avg_V : Subsystem  TreatAsAtomicUnit=on
  Bat_cap_Ah : Subsystem  TreatAsAtomicUnit=on
  Bat_power_max_kW : Subsystem  TreatAsAtomicUnit=on
  Bat_power_min_kW : Subsystem  TreatAsAtomicUnit=on
  DCAC_eff : Subsystem  TreatAsAtomicUnit=on
  DCAC效率 : Constant  Value=DCAC_eff
  FC_power-MAX : Constant  Value=FC_power_max_kW
  FC_power-MIN1 : Constant  Value=FC_power_min_kW
  FC_power_max_kW : Subsystem  TreatAsAtomicUnit=on
  FC_power_min_kW : Subsystem  TreatAsAtomicUnit=on
  MC_power_req_kW : Subsystem  TreatAsAtomicUnit=on
  Mux1 : Mux  Inputs=15
  Mux2 : Mux  Inputs=6
  S-Function1 : S-Function  FunctionName=Fun_EF  SFunctionDeploymentMode=off  EnableBusSupport=off
  Scope : Scope
  Sum2 : Sum  Inputs=-+  InputSameDT=on  SaturateOnIntegerOverflow=on  OutDataTypeStr=Inherit: Same as first input
  X_r_km : Subsystem  TreatAsAtomicUnit=on
  alpha : Subsystem  TreatAsAtomicUnit=on
  总行驶里程(km) : Constant  Value=Trip_distance_total_km
  权值 : Constant  Value=alpha
  电池容量 : Constant  Value=Bat_ori_cap_max_Ah
  电池组平均电压 : Constant  Value=Bat_U_avg_V
  等效因子 : ToWorkspace  VariableName=EMS_EF  SampleTime=-1
  TO SQP : Outport
  tag scope: EF=global
  wires:
  [Bat_SOC] -> Bat_SOC/1(In1)
  .2/1 -> Bat_SOC/Enable
  [PS_power_req_kW] -> MC_power_req_kW/1(In1)
  .3/1 -> MC_power_req_kW/Enable
  .6/1 -> DCAC_eff/Enable
  DCAC效率/1 -> DCAC_eff/1(In1)
  Bat_SOC/1(Out1) -> Mux2/4, Mux1/1
  MC_power_req_kW/1(Out1) -> Mux1/2
  Mux1/1 -> TO SQP/1
  [Trip_distance_travelled_km] -> Sum2/1
  .1/1 -> X_r_km/Enable
  X_r_km/1(Out1) -> Mux2/2, Mux1/3
  Sum2/1 -> X_r_km/1(In1)
  总行驶里程(km)/1 -> Sum2/2
  [Trip_distance_EV_km] -> "    DC_type"/1(In1)
  .10/1 -> "    DC_type"/Enable
  权值/1 -> alpha/1(In1)
  alpha/1(Out1) -> Mux1/5
  .4/1 -> alpha/Enable
  DCAC_eff/1(Out1) -> Mux1/6
  .7/1 -> Bat_SOC_min/Enable
  Bat_SOC-MIN/1 -> Bat_SOC_min/1(In1)
  .12/1 -> Bat_SOC_max/Enable
  Bat_SOC-MAX/1 -> Bat_SOC_max/1(In1)
  Bat_SOC_max/1(Out1) -> Mux1/8
  电池容量/1 -> Bat_cap_Ah/1(In1)
  .13/1 -> Bat_cap_Ah/Enable
  Bat_cap_Ah/1(Out1) -> Mux1/10
  Bat_SOC_min/1(Out1) -> Mux2/5, Mux1/7
  .14/1 -> Bat_SOC_ref/Enable
  [Bat_SOC_ref] -> Bat_SOC_ref/1(In1)
  Bat_SOC_ref/1(Out1) -> Mux2/6, Mux1/9
  .5/1 -> Bat_power_min_kW/Enable
  .8/1 -> Bat_power_max_kW/Enable
  [Bat_power_chg_max_kW] -> Bat_power_min_kW/1(In1)
  [Bat_power_dis_max_kW] -> Bat_power_max_kW/1(In1)
  .9/1 -> FC_power_min_kW/Enable
  .11/1 -> FC_power_max_kW/Enable
  FC_power-MIN1/1 -> FC_power_min_kW/1(In1)
  FC_power-MAX/1 -> FC_power_max_kW/1(In1)
  Bat_power_min_kW/1(Out1) -> Mux1/12
  Bat_power_max_kW/1(Out1) -> Mux1/13
  FC_power_min_kW/1(Out1) -> Mux1/14
  FC_power_max_kW/1(Out1) -> Mux1/15
  电池组平均电压/1 -> Bat_U_avg_V/1(In1)
  .15/1 -> Bat_U_avg_V/Enable
  Bat_U_avg_V/1(Out1) -> Mux1/11
  [Bat_power_ref_kW] -> Mux2/1
  "    DC_type"/1(Out1) -> Mux2/3, Mux1/4
  Mux2/1 -> S-Function1/1
  S-Function1/1 -> [EF], Scope/1, 等效因子/1

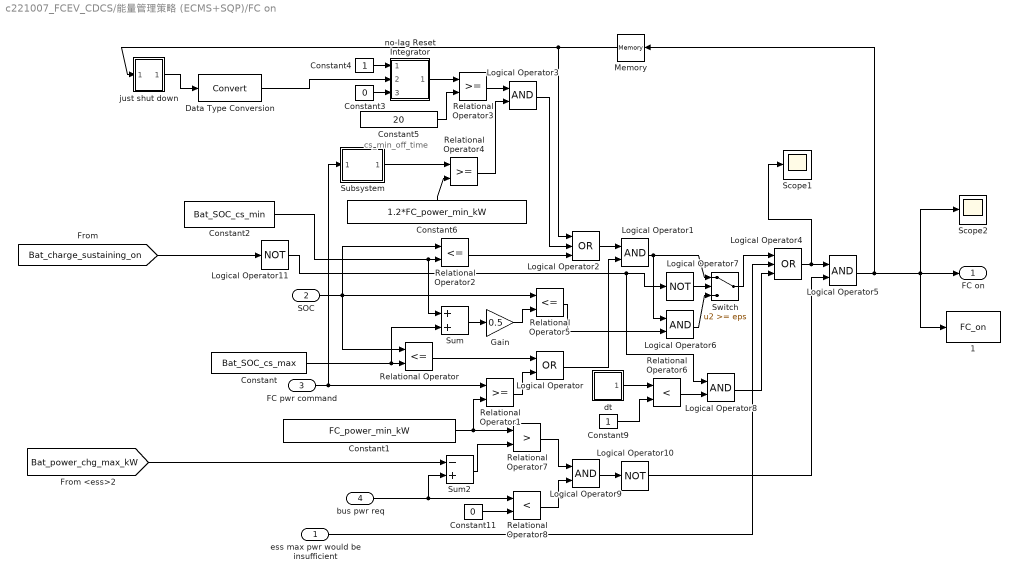
== system c221007_FCEV_CDCS/能量管理策略 (ECMS+SQP)/FC on ==
  note: cs_min_off_time
  ess max pwr would be insufficient : Inport
  SOC : Inport  Port=2
  FC pwr command : Inport  Port=3
  bus pwr req : Inport  Port=4
  "  1" : ToWorkspace  VariableName=FC_on  SampleTime=-1
  Constant : Constant  Value=Bat_SOC_cs_max
  Constant1 : Constant  Value=FC_power_min_kW
  Constant11 : Constant  Value=0
  Constant2 : Constant  Value=Bat_SOC_cs_min
  Constant3 : Constant  Value=0
  Constant4 : Constant
  Constant5 : Constant  Value=20
  Constant6 : Constant  Value=1.2*FC_power_min_kW
  Constant9 : Constant
  Data Type Conversion : DataTypeConversion  SaturateOnIntegerOverflow=off  RndMeth=Floor
  Gain : Gain  Gain=0.5  SaturateOnIntegerOverflow=on  OutDataTypeStr=Inherit: Same as input  ParamDataTypeStr=Inherit: Same as input
  Logical Operator : Logic  Operator=OR
  Logical Operator{1,3,6,8..9} (5 alike) : Logic
  Logical Operator10 : Logic  Operator=NOT
  Logical Operator11 : Logic  Operator=NOT  Inputs=1  OutDataTypeStr=boolean
  Logical Operator2 : Logic  Operator=OR  Inputs=3
  Logical Operator4 : Logic  Operator=OR  Inputs=3
  Logical Operator5 : Logic  OutDataTypeStr=boolean
  Logical Operator7 : Logic  Operator=NOT  Inputs=1  OutDataTypeStr=boolean
  Memory : Memory  InheritSampleTime=on
  Relational Operator : RelationalOperator  Operator=<=
  Relational Operator1 : RelationalOperator
  Relational Operator2 : RelationalOperator  Operator=<=
  Relational Operator3 : RelationalOperator
  Relational Operator4 : RelationalOperator
  Relational Operator5 : RelationalOperator  Operator=<=
  Relational Operator6 : RelationalOperator  Operator=<
  Relational Operator7 : RelationalOperator  Operator=>
  Relational Operator8 : RelationalOperator  Operator=<
  Scope1 : Scope
  Scope2 : Scope
  Subsystem : Subsystem  mask(Running Average){n=5}
      mask prompts: n "Averaging Time (s)"
      mask help: Running Average
      mask Help: Output is the average of the last (Averaging Time) seconds of input.
      mask Display: disp('Running\nAverage')
  Sum : Sum  InputSameDT=on  SaturateOnIntegerOverflow=on  OutDataTypeStr=Inherit: Same as first input
  Sum2 : Sum  Inputs=-+  InputSameDT=on  SaturateOnIntegerOverflow=on  OutDataTypeStr=Inherit: Same as first input
  Switch : Switch  Threshold=eps
  dt : Subsystem
  just shut down : Subsystem
  no-lag Reset Integrator : Subsystem  mask(No-lag Reset Integrator){initval=0}
      mask prompts: initval "Initial Value"
      mask help: No-lag Reset Integrator
      mask Help: Integrates first input using Euler technique.\nAt the time step that input 2 <> zero,\noutput is reset to input 3.
      mask Display: disp('1/s\nw/ reset\nno lag')
  FC on : Outport
  wires:
  Constant1/1 -> Relational Operator7/1, Relational Operator1/2
  Relational Operator8/1 -> Logical Operator9/2
  Relational Operator7/1 -> Logical Operator9/1
  Logical Operator10/1 -> Logical Operator5/2
  Logical Operator9/1 -> Logical Operator10/1
  Logical Operator/1 -> Logical Operator1/2
  Sum2/1 -> Relational Operator7/2
  bus pwr req/1 -> Sum2/2, Relational Operator8/1
  Constant11/1 -> Relational Operator8/2
  Relational Operator/1 -> Logical Operator/1
  Relational Operator2/1 -> Logical Operator2/3
  Relational Operator5/1 -> Logical Operator6/2
  ess max pwr would be insufficient/1 -> Logical Operator4/2
  FC pwr command/1 -> Subsystem/1(in_1), Relational Operator1/1
  Relational Operator1/1 -> Logical Operator/2
  SOC/1 -> Relational Operator2/1, Relational Operator/1, Relational Operator5/1
  Logical Operator2/1 -> Logical Operator1/1
  Logical Operator3/1 -> Logical Operator2/2
  Subsystem/1(out_1) -> Relational Operator4/1
  Relational Operator4/1 -> Logical Operator3/2
  Constant6/1 -> Relational Operator4/2
  Constant4/1 -> no-lag Reset Integrator/1(in_1)
  Constant3/1 -> no-lag Reset Integrator/3(in_3)
  no-lag Reset Integrator/1(out_1) -> Relational Operator3/1
  Relational Operator3/1 -> Logical Operator3/1
  Constant5/1 -> Relational Operator3/2
  Memory/1 -> Logical Operator2/1, just shut down/1(state)
  Constant2/1 -> Relational Operator2/2, Sum/1
  Constant/1 -> Relational Operator/2, Sum/2
  Sum/1 -> Gain/1
  Gain/1 -> Relational Operator5/2
  Logical Operator7/1 -> Switch/2
  Logical Operator6/1 -> Switch/3
  Logical Operator1/1 -> Switch/1, Logical Operator6/1
  Switch/1 -> Logical Operator4/1
  Logical Operator11/1 -> Logical Operator7/1, Logical Operator8/1
  Logical Operator8/1 -> Logical Operator4/3
  dt/1(out_1) -> Relational Operator6/1
  Constant9/1 -> Relational Operator6/2
  Relational Operator6/1 -> Logical Operator8/2
  just shut down/1(trigger) -> Data Type Conversion/1
  Data Type Conversion/1 -> no-lag Reset Integrator/2(in_2)
  Logical Operator4/1 -> Logical Operator5/1, Scope1/1
  Logical Operator5/1 -> "  1"/1, Scope2/1, FC on/1, Memory/1
  [Bat_charge_sustaining_on] -> Logical Operator11/1
  [Bat_power_chg_max_kW] -> Sum2/1

== system c221007_FCEV_CDCS/能量管理策略 (ECMS+SQP)/FC pwr command, w// limits enforced ==
  note: 电池放电功率能满足整车需求功率
      | 以及SOC>=SOCmin, and输出为1
  ess max pwr would be insufficient : Inport
  SOC : Inport  Port=2
  FC pwr command : Inport  Port=3
  Constant1 : Constant  Value=Bat_SOC_min
  Logical Operator : Logic  OutDataTypeStr=boolean
  Logical Operator1 : Logic  Operator=NOT  Inputs=1
  MinMax : MinMax  Function=max  Inputs=2  InputSameDT=on  SaturateOnIntegerOverflow=on
  MinMax1 : MinMax  Inputs=2  InputSameDT=on  SaturateOnIntegerOverflow=on
  Relational Operator : RelationalOperator
  Switch : Switch  Threshold=eps
  cs_max_power : Constant  Value=FC_power_max_kW
  cs_min_power : Constant  Value=FC_power_min_kW
  limited FC pwr command (W) : Outport
  wires:
  FC pwr command/1 -> MinMax/1
  cs_min_power/1 -> Switch/1, MinMax/2
  cs_max_power/1 -> MinMax1/1
  MinMax/1 -> MinMax1/2
  Switch/1 -> limited FC pwr command (W)/1
  Constant1/1 -> Relational Operator/2
  Logical Operator/1 -> Switch/2
  SOC/1 -> Relational Operator/1
  Relational Operator/1 -> Logical Operator/2
  Logical Operator1/1 -> Logical Operator/1
  ess max pwr would be insufficient/1 -> Logical Operator1/1
  MinMax1/1 -> Switch/3

== system c221007_FCEV_CDCS/能量管理策略 (ECMS+SQP)/SQP ==
  From Collection : Inport
  Demux1 : Demux  Outputs=2
      settings: DisplayOption=none
  Power limitation : Subsystem
  S-Function1 : S-Function  FunctionName=ENERGY_MANAGE_SQP  SFunctionDeploymentMode=off  EnableBusSupport=off
  Pwr_b : Outport
  Pwr_fc : Outport  Port=2
  tag scope: Bat_power_ref_kW=global, FC_power_ref_kW=global
  wires:
  From Collection/1 -> S-Function1/1
  S-Function1/1 -> Demux1/1
  Demux1/1 -> [Bat_power_ref_kW], Pwr_b/1
  Demux1/2 -> [FC_power_ref_kW], Pwr_fc/1

== system c221007_FCEV_CDCS/行驶工况相关/Custom Neural Network ==
  Input : Inport  PortDimensions=3
      mask Display: e = 0.06;c1 = [120 230 180]/255;c2 = ([120 230 180]+0)/(256+128);c3 = ([120 230 180]+128)/(256+128);patch([0 1 1 0],[0 0 1 1],c1);patch([0 1 1 1-e 1-e 0+e],[0 0 1 1-e 0+e 0+e],c2);patch([0 0 1 1-e 0+e 0+e],[0 1 1 1-e 1-e 0+e],c3);plot([0 1 1 0 0],[0 0 1 1 0]);
  Layer 1 : Subsystem
      mask Display: e = 0.06;c1 = [120 150 230]/255;c2 = ([120 150 230]+0)/383;c3 = ([120 150 230]+128)/383;patch([0 1 1 0],[0 0 1 1],c1);patch([0 1 1 1-e 1-e 0+e],[0 0 1 1-e 0+e 0+e],c2);patch([0 0 1 1-e 0+e 0+e],[0 1 1 1-e 1-e 0+e],c3);plot([0 1 1 0 0],[0 0 1 1 0]);
  Layer 2 : Subsystem
      mask Display: e = 0.06;c1 = [120 150 230]/255;c2 = ([120 150 230]+0)/383;c3 = ([120 150 230]+128)/383;patch([0 1 1 0],[0 0 1 1],c1);patch([0 1 1 1-e 1-e 0+e],[0 0 1 1-e 0+e 0+e],c2);patch([0 0 1 1-e 0+e 0+e],[0 1 1 1-e 1-e 0+e],c3);plot([0 1 1 0 0],[0 0 1 1 0]);
  Process Input 1 : Subsystem
      mask Display: e = 0.06;c1 = [120 150 230]/255;c2 = ([120 150 230]+0)/383;c3 = ([120 150 230]+128)/383;patch([0 1 1 0],[0 0 1 1],c1);patch([0 1 1 1-e 1-e 0+e],[0 0 1 1-e 0+e 0+e],c2);patch([0 0 1 1-e 0+e 0+e],[0 1 1 1-e 1-e 0+e],c3);plot([0 1 1 0 0],[0 0 1 1 0]);
  Process Output 1 : Subsystem
      mask Display: e = 0.06;c1 = [120 150 230]/255;c2 = ([120 150 230]+0)/383;c3 = ([120 150 230]+128)/383;patch([0 1 1 0],[0 0 1 1],c1);patch([0 1 1 1-e 1-e 0+e],[0 0 1 1-e 0+e 0+e],c2);patch([0 0 1 1-e 0+e 0+e],[0 1 1 1-e 1-e 0+e],c3);plot([0 1 1 0 0],[0 0 1 1 0]);
  Output : Outport  InitialOutput=[0;0;0]
      mask Display: e = 0.06;c1 = [120 230 180]/255;c2 = ([120 230 180]+0)/(256+128);c3 = ([120 230 180]+128)/(256+128);patch([0 1 1 0],[0 0 1 1],c1);patch([0 1 1 1-e 1-e 0+e],[0 0 1 1-e 0+e 0+e],c2);patch([0 0 1 1-e 0+e 0+e],[0 1 1 1-e 1-e 0+e],c3);plot([0 1 1 0 0],[0 0 1 1 0]);
  wires:
  Input/1 -> Process Input 1/1(x)
  Process Output 1/1(y) -> Output/1
  Process Input 1/1(p) -> Layer 1/1("p{1}")
  Layer 1/1("a{1}") -> [feedback1]
  [feedback1] -> Layer 2/1("a{1} ")
  Layer 2/1("a{2}") -> Process Output 1/1(a)

== system c221007_FCEV_CDCS/车轮模型/Interia torque ==
  note: This block computes the torque required to overcome the inertia of the
      | wheels and axle.
  车轮线速度 m/s : Inport
  Add : Sum  Inputs=+-
  Constant : Constant  Value=Veh_wheel_inertia
  Constant2 : Constant  Value=0
  Divide : Product  Inputs=**
  Memory : Memory  InheritSampleTime=on
  Switch : Switch  Criteria=u2 > Threshold  SaturateOnIntegerOverflow=off  InputSameDT=off
  axle input speed (rad/s) : Gain  Gain=1/Veh_wheel_radius_m
  inertia torque (Nm) : Outport  InitialOutput=0
  wires:
  Switch/1 -> Divide/1
  Constant/1 -> Divide/2
  Memory/1 -> Add/2
  axle input speed (rad/s)/1 -> Memory/1, Add/1
  车轮线速度 m/s/1 -> axle input speed (rad/s)/1
  Divide/1 -> inertia torque (Nm)/1
  Add/1 -> Switch/1, Switch/2
  Constant2/1 -> Switch/3

== system c221007_FCEV_CDCS/车轮模型/Interia torque1 ==
  note: This block computes the torque required to overcome the inertia of the
      | wheels and axle.
  车轮线速度 m/s : Inport
  Add : Sum  Inputs=+-
  Add1 : Sum  Inputs=+-
  Clock : Clock
  Constant : Constant  Value=Veh_wheel_inertia
  Constant2 : Constant  Value=0
  Divide : Product  Inputs=**/
  Memory : Memory  InheritSampleTime=on
  Memory1 : Memory  InheritSampleTime=on
  Saturation : Saturate  UpperLimit=1.1  LowerLimit=0.9
  Switch : Switch  SaturateOnIntegerOverflow=off  InputSameDT=off
  axle input speed (rad/s) : Gain  Gain=1/Veh_wheel_radius_m
  inertia torque (Nm) : Outport  InitialOutput=0
  wires:
  Switch/1 -> Divide/1
  Add/1 -> Switch/2, Switch/3
  Constant/1 -> Divide/2
  Memory1/1 -> Add1/2
  Clock/1 -> Memory1/1, Add1/1
  Memory/1 -> Add/2
  axle input speed (rad/s)/1 -> Memory/1, Add/1
  Constant2/1 -> Switch/1
  Add1/1 -> Saturation/1
  Saturation/1 -> Divide/3
  车轮线速度 m/s/1 -> axle input speed (rad/s)/1
  Divide/1 -> inertia torque (Nm)/1

== system c221007_FCEV_CDCS/车轮模型/Regenerative energy compute ==
  motor brk force : Inport
  spd : Inport  Port=2
  spd2 : Inport  Port=3
  Add : Sum
  Divide : Product  Inputs=*/
  Gain1 : Gain  Gain=-1
  Memory : Memory  InitialCondition=0.1  InheritSampleTime=on
  Product : Product  RndMeth=Zero
  Saturation : Saturate  UpperLimit=-0.1  LowerLimit=-1000000
  To Workspace : ToWorkspace  VariableName=Energy_regenerative_brk_percent  SaveFormat=Timeseries  SampleTime=-1
  Ws->kWh : Gain  Gain=1/(1000*3600)
  compute of the brk energy : Subsystem
  wires:
  [Veh_force_brk_req_N] -> Product/2
  spd2/1 -> Product/1
  compute of the brk energy/1("regenerative brk energy kwh ") -> Divide/1
  Divide/1 -> To Workspace/1
  motor brk force/1 -> compute of the brk energy/1(motor brk force in front wheel N)
  spd/1 -> compute of the brk energy/2(wheel linear spd m/s)
  Saturation/1 -> Gain1/1
  Gain1/1 -> Ws->kWh/1
  Ws->kWh/1 -> Divide/2
  Add/1 -> Memory/1, Saturation/1
  Memory/1 -> Add/2
  Product/1 -> Add/1

== system c221007_FCEV_CDCS/车轮模型/Tire slip model ==
  In1 : Inport
  Add : Sum
  Constant : Constant  Value=Veh_gravity_acc_ms2
  Constant1 : Constant  Value=Veh_mass_curb_kg
  Constant2 : Constant  Value=Veh_mass_cargo_kg
  Constant3 : Constant  Value=Veh_wt_frac_front
  Constant4 : Constant  Value=Road_u
  Memory : Memory  InheritSampleTime=on
  MinMax : MinMax  Inputs=2  SampleTime=0
  Product : Product  Inputs=4  RndMeth=Zero
  dri_force available in front wheel n : Outport
  wires:
  Constant1/1 -> Add/1
  Constant2/1 -> Add/2
  Add/1 -> Product/3
  Constant3/1 -> Product/2
  Constant/1 -> Product/1
  Constant4/1 -> Product/4
  Product/1 -> Memory/1
  In1/1 -> MinMax/1
  MinMax/1 -> dri_force available in front wheel n/1
  Memory/1 -> MinMax/2

== system c221007_FCEV_CDCS/车轮模型/Tire slip model1 ==
  In1 : Inport
  Add : Sum
  Constant : Constant  Value=Veh_gravity_acc_ms2
  Constant1 : Constant  Value=Veh_mass_curb_kg
  Constant2 : Constant  Value=Veh_mass_cargo_kg
  Constant3 : Constant  Value=Veh_wt_frac_front
  Constant4 : Constant  Value=Road_u
  Gain1 : Gain  Gain=-1
  Memory : Memory  InheritSampleTime=on
  MinMax : MinMax  Function=max  Inputs=2  SampleTime=0
  Product : Product  Inputs=4  RndMeth=Zero
  brk_force available in front wheel n : Outport
  wires:
  Constant1/1 -> Add/1
  Constant2/1 -> Add/2
  Add/1 -> Product/3
  Constant3/1 -> Product/2
  Constant/1 -> Product/1
  Constant4/1 -> Product/4
  In1/1 -> MinMax/1
  MinMax/1 -> brk_force available in front wheel n/1
  Memory/1 -> MinMax/2
  Product/1 -> Gain1/1
  Gain1/1 -> Memory/1

== system c221007_FCEV_CDCS/驱动电机模型/Brake torque_limited ==
  tor_req nm : Inport
  mc spd rpm : Inport  Port=2
  1-D Lookup Table : Lookup_n-D  NumberOfTableDimensions=1  BreakpointsForDimension1=MC_ori_spd_rpm  Table=MC_ori_trq_brk_max_Nm  RndMeth=Simplest
  MinMax : MinMax  Function=max  Inputs=2
  limted mc torque nm : Outport
  wires:
  tor_req nm/1 -> MinMax/1
  mc spd rpm/1 -> 1-D Lookup Table/1
  1-D Lookup Table/1 -> MinMax/2
  MinMax/1 -> limted mc torque nm/1

== system c221007_FCEV_CDCS/驱动电机模型/Drive torque_limited ==
  tor_req nm : Inport
  mc spd rpm : Inport  Port=2
  1-D Lookup Table : Lookup_n-D  NumberOfTableDimensions=1  BreakpointsForDimension1=MC_ori_spd_rpm  Table=MC_ori_trq_dri_max_Nm  RndMeth=Simplest
  MinMax : MinMax  Inputs=2
  limted mc torque nm : Outport
  wires:
  tor_req nm/1 -> MinMax/1
  mc spd rpm/1 -> 1-D Lookup Table/1
  1-D Lookup Table/1 -> MinMax/2
  MinMax/1 -> limted mc torque nm/1

== system c221007_FCEV_CDCS/驱动电机模型/Inertia torque ==
  motor spd rpm : Inport
  Derivative : Derivative
  Gain1 : Gain  Gain=MC_inertia
  rpm->rad/s : Gain  Gain=2*pi/60
  Out1 : Outport
  wires:
  Derivative/1 -> Gain1/1
  Gain1/1 -> Out1/1
  rpm->rad/s/1 -> Derivative/1
  motor spd rpm/1 -> rpm->rad/s/1

== system c221007_FCEV_CDCS/驱动电机模型/Inertia torque1 ==
  motor spd rpm : Inport
  Derivative : Derivative
  Gain1 : Gain  Gain=MC_inertia
  rpm->rad/s : Gain  Gain=2*pi/60
  Out1 : Outport
  wires:
  Derivative/1 -> Gain1/1
  Gain1/1 -> Out1/1
  rpm->rad/s/1 -> Derivative/1
  motor spd rpm/1 -> rpm->rad/s/1

== system c221007_FCEV_CDCS/驱动电机模型/nm tor per pwr w input ==
  dri nm : Inport
  pwr dri kW : Inport  Port=2
  Add4 : Sum
  Constant : Constant  Value=eps
  Constant1 : Constant  Value=0
  Constant2 : Constant  Value=inf
  Divide : Product  Inputs=*/
  Relational Operator : RelationalOperator  Operator=~=  OutDataTypeStr=boolean  InputSameDT=off
  Switch : Switch  Threshold=eps  SaturateOnIntegerOverflow=off  InputSameDT=off
  kW->W : Gain  Gain=1000
  tor per pwr : Outport
  wires:
  Constant/1 -> Add4/2
  Add4/1 -> Divide/2
  dri nm/1 -> Divide/1
  Divide/1 -> Switch/1
  Constant1/1 -> Relational Operator/2
  Relational Operator/1 -> Switch/2
  Constant2/1 -> Switch/3
  pwr dri kW/1 -> kW->W/1
  Switch/1 -> tor per pwr/1
  kW->W/1 -> Add4/1, Relational Operator/1

== system c221007_FCEV_CDCS/驱动电机模型/nm tor per pwr w input1 ==
  pwr brk kW : Inport
  brk nm : Inport  Port=2
  Add4 : Sum
  Constant : Constant  Value=eps
  Constant1 : Constant  Value=0
  Constant2 : Constant  Value=inf
  Divide : Product  Inputs=*/
  Gain1 : Gain  Gain=-1
  Gain2 : Gain  Gain=-1000
  Relational Operator : RelationalOperator  Operator=~=  OutDataTypeStr=boolean  InputSameDT=off
  Switch : Switch  Threshold=eps  SaturateOnIntegerOverflow=off  InputSameDT=off
  tor per pwr : Outport
  wires:
  Gain2/1 -> Relational Operator/1, Add4/1
  Switch/1 -> tor per pwr/1
  Constant2/1 -> Switch/3
  Relational Operator/1 -> Switch/2
  Constant1/1 -> Relational Operator/2
  Divide/1 -> Switch/1
  Gain1/1 -> Divide/1
  Add4/1 -> Divide/2
  Constant/1 -> Add4/2
  pwr brk kW/1 -> Gain2/1
  brk nm/1 -> Gain1/1

== system c221007_FCEV_CDCS/驱动电机模型/rotor available brake torque nm ==
  tor per pwr : Inport
  pwr available kW : Inport  Port=2
  Constant : Constant  Value=inf
  Constant1 : Constant  Value=0
  Product : Product  RndMeth=Zero
  Relational Operator : RelationalOperator  Operator=~=  OutDataTypeStr=boolean  InputSameDT=off
  Switch : Switch  Threshold=0.3  SaturateOnIntegerOverflow=off  InputSameDT=off
  kW->W : Gain  Gain=1000
  tor avaible nm : Outport
  wires:
  Switch/1 -> tor avaible nm/1
  Constant1/1 -> Switch/3
  Relational Operator/1 -> Switch/2
  Constant/1 -> Relational Operator/2
  Product/1 -> Switch/1
  tor per pwr/1 -> Product/1, Relational Operator/1
  kW->W/1 -> Product/2
  pwr available kW/1 -> kW->W/1

== system c221007_FCEV_CDCS/驱动电机模型/rotor available drive torque nm ==
  tor per pwr : Inport
  pwr available kW : Inport  Port=2
  Constant : Constant  Value=inf
  Constant1 : Constant  Value=0
  Product : Product  RndMeth=Zero
  Relational Operator : RelationalOperator  Operator=~=  OutDataTypeStr=boolean  InputSameDT=off
  Switch : Switch  Threshold=0.3  SaturateOnIntegerOverflow=off  InputSameDT=off
  kW->W : Gain  Gain=1000
  tor avaible nm : Outport
  wires:
  Product/1 -> Switch/1
  Constant/1 -> Relational Operator/2
  Relational Operator/1 -> Switch/2
  Constant1/1 -> Switch/3
  tor per pwr/1 -> Product/1, Relational Operator/1
  Switch/1 -> tor avaible nm/1
  kW->W/1 -> Product/2
  pwr available kW/1 -> kW->W/1
